simulink model "integrator"  (R2025a)
settings: Solver=FixedStepDiscrete  StartTime=0.0  StopTime=1000/100000000  RelTol=1e-3
undefined symbols (not defined in the file): DiscIntNeverNeededParam
libraries: simulink x1
settings Model: Creator=Luiz  LastModifiedBy=Luiz

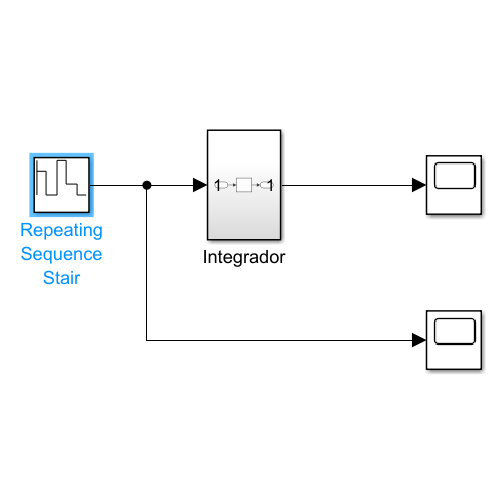
[thumbnail: Simulink's stored preview of the top-level diagram]
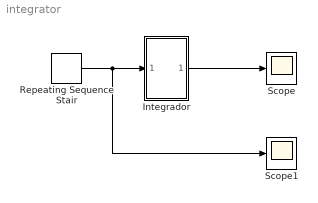
== system integrator ==
  Integrador : Subsystem
  Repeating Sequence Stair : simulink/Sources/Repeating Sequence Stair  OutValues=[3 1 4 2 1].'  tsamp=-1  OutMin=[]  OutMax=[]  OutDataTypeStr=double  OutputDataTypeScalingMode=double  OutDataType=fixdt(0,8)  ConRadixGroup=Best Precision: Vector-wise  OutScaling=2^-12
  Scope : Scope
      settings: ActiveDisplayYMinimum=-5.864285714285722E-7  ActiveDisplayYMaximum=2.5970401785714289E-6
  Scope1 : Scope
      settings: ActiveDisplayYMinimum=0.24568622256738726  ActiveDisplayYMaximum=4.5867799725673883
  wires:
  Repeating Sequence Stair/1 -> Scope1/1, Integrador/1(In1)
  Integrador/1(Out1) -> Scope/1

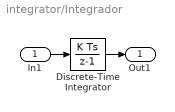
== system integrator/Integrador ==
  In1 : Inport
  Discrete-Time Integrator : DiscreteIntegrator  SampleTime=100/100000000  ICPrevOutput=DiscIntNeverNeededParam  ICPrevScaledInput=DiscIntNeverNeededParam
  Out1 : Outport
  wires:
  In1/1 -> Discrete-Time Integrator/1
  Discrete-Time Integrator/1 -> Out1/1
